simulink model "Syn_Leader_Follower_ext2"  (R2021a)
settings: Solver=VariableStepAuto  StartTime=0.0  StopTime=5  RelTol=1e-3
settings Model: Creator=JianFongLee  LastModifiedBy=JianFongLee

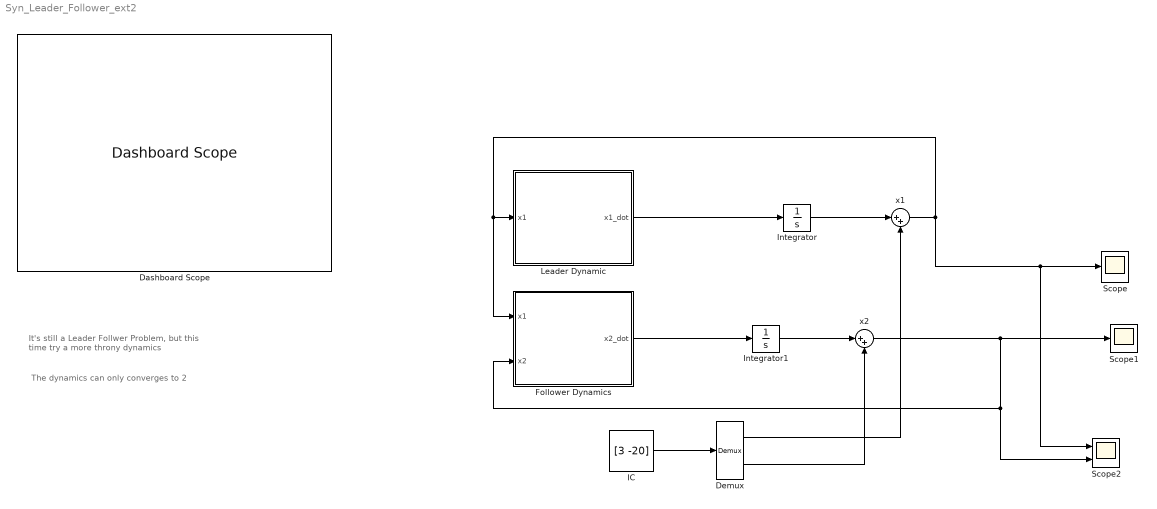
== system Syn_Leader_Follower_ext2 ==
  note: The dynamics can only converges to 2
  note: It's still a Leader Follwer Problem,
      | but this time try a more throny dynamics
  Dashboard Scope : DashboardScope
  Demux : Demux  Outputs=2
      settings: DisplayOption=none
  Follower Dynamics : MATLAB Function  TreatAsAtomicUnit=on
  IC : Constant  Value=[3 -20]
  Integrator : Integrator
  Integrator1 : Integrator
  Leader Dynamic : MATLAB Function  TreatAsAtomicUnit=on
  Scope : Scope
  Scope1 : Scope
  Scope2 : Scope  NumInputPorts=2
  x1 : Sum  Inputs=|++
  x2 : Sum  Inputs=|++
  wires:
  Leader Dynamic/1(x1_dot) -> Integrator/1
  Integrator/1 -> x1/1
  x1/1 -> Scope2/1, Scope/1, Follower Dynamics/1(x1), Leader Dynamic/1(x1)
  Follower Dynamics/1(x2_dot) -> Integrator1/1
  IC/1 -> Demux/1
  Demux/1 -> x1/2
  Integrator1/1 -> x2/1
  Demux/2 -> x2/2
  x2/1 -> Scope2/2, Follower Dynamics/2(x2), Scope1/1

== matlab function Syn_Leader_Follower_ext2/Leader Dynamic ==
  data: x1 input; x1_dot output
function x1_dot = fcn(x1)
 
%%% System leader
x1_dot = x1*(x1-2)*(x1-5);
%%% This system converges to 2 for x>0 && x<5,
%%% 0 dynamics for x =0,5 ,
%%% and blows up for the rest states.

%%% It's an unstable system basically
%%% So, as a leader, its IC should be within 0 to 5,
%%% it needs to be converges itself
end

== matlab function Syn_Leader_Follower_ext2/Follower Dynamics ==
  data: x1 input; x2_dot output; x2 input
function x2_dot = fcn(x1,x2)
 
%%% System follower, comprising u to syn with x1
ux1 = 4/3*x1^3 - 7*x1^2 +10*x1;
ux2 = 4/3*x2^3 - 7*x2^2 +10*x2;
u = ux1 - ux2;

x2_dot = x2*(x2-2)*(x2-5) + u;
%%% With the same dynamics of x1 except u is employed,
%%% so it would follow where x1 ends up in this case.

%%% Let its IC be in the range of going nuts,
%%% and see how it follows the leader to converge.
end
